simulink model "control1"  (R2024b)
settings: Solver=ode4  StartTime=0.0  StopTime=4.0  FixedStep=1e-3  RelTol=1e-3
settings Model: Creator=mehmetcanevi  LastModifiedBy=mehmetcanevi

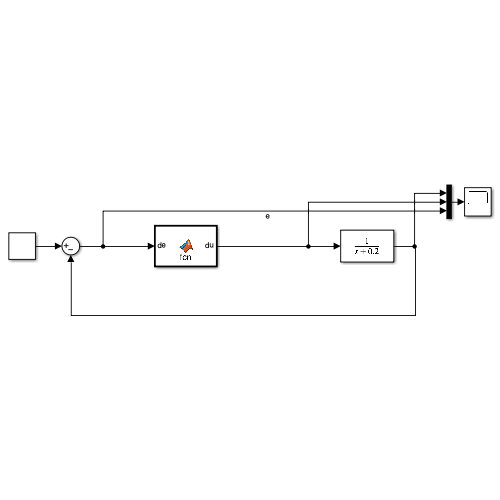
[thumbnail: Simulink's stored preview of the top-level diagram]
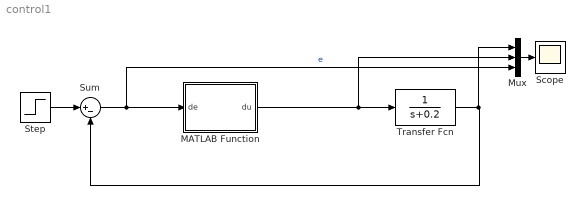
== system control1 ==
  MATLAB Function : MATLAB Function  TreatAsAtomicUnit=on
  Mux : Mux  Inputs=3
  Scope : Scope
  Step : Step  SampleTime=0
  Sum : Sum  Inputs=|+-
  Transfer Fcn : TransferFcn  Denominator=[1 0.2]
  wires:
  Step/1 -> Sum/1
  Transfer Fcn/1 -> Mux/1, Sum/2
  Sum/1 -> Mux/3, MATLAB Function/1(de)  "e"
  Mux/1 -> Scope/1
  MATLAB Function/1(du) -> Mux/2, Transfer Fcn/1

== matlab function control1/MATLAB Function ==
  data: de input; du output
function du = fcn(de)
L=0.25;
H=10*L;
    if de<-L
        du = -H;
    elseif de>=-L && de<=L
        du=(H/L)*de;
    else
        du = H;
    end
end
